simulink model "prueba_cinematica"  (Simulink 7.6)
settings: Solver=ode45  StartTime=0.0  StopTime=10.0  RelTol=1e-3
undefined symbols (not defined in the file or in its folder): phi0, psi0, theta0, x0, y0, z0
settings Model: Creator=pater  LastModifiedBy=pater

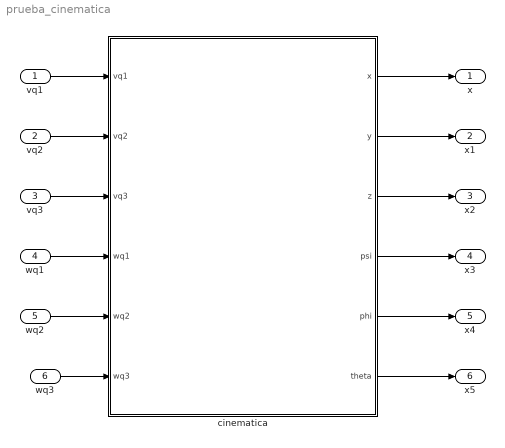
== system prueba_cinematica ==
  vq1 : Inport
  vq2 : Inport  Port=2
  vq3 : Inport  Port=3
  wq1 : Inport  Port=4
  wq2 : Inport  Port=5
  wq3 : Inport  Port=6
  cinematica : Subsystem
  x : Outport
  x1 : Outport  Port=2
  x2 : Outport  Port=3
  x3 : Outport  Port=4
  x4 : Outport  Port=5
  x5 : Outport  Port=6
  wires:
  vq1/1 -> cinematica/1(vq1)
  vq2/1 -> cinematica/2(vq2)
  vq3/1 -> cinematica/3(vq3)
  wq1/1 -> cinematica/4(wq1)
  wq2/1 -> cinematica/5(wq2)
  wq3/1 -> cinematica/6(wq3)
  cinematica/6(theta) -> x5/1
  cinematica/5(phi) -> x4/1
  cinematica/4(psi) -> x3/1
  cinematica/3(z) -> x2/1
  cinematica/2(y) -> x1/1
  cinematica/1(x) -> x/1

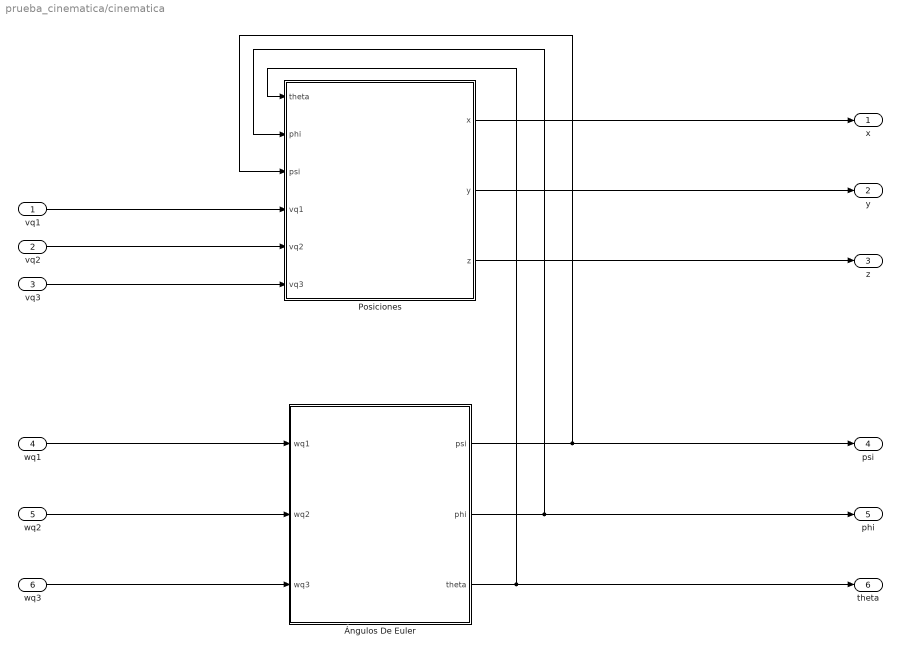
== system prueba_cinematica/cinematica ==
  vq1 : Inport
  vq2 : Inport  Port=2
  vq3 : Inport  Port=3
  wq1 : Inport  Port=4
  wq2 : Inport  Port=5
  wq3 : Inport  Port=6
  Posiciones : Subsystem
  Ángulos De Euler : Subsystem
  x : Outport
  y : Outport  Port=2
  z : Outport  Port=3
  psi : Outport  Port=4
  phi : Outport  Port=5
  theta : Outport  Port=6
  wires:
  Posiciones/1(x) -> x/1
  Posiciones/2(y) -> y/1
  Posiciones/3(z) -> z/1
  Ángulos De Euler/1(psi) -> psi/1, Posiciones/3(psi)
  Ángulos De Euler/2(phi) -> phi/1, Posiciones/2(phi)
  Ángulos De Euler/3(theta) -> theta/1, Posiciones/1(theta)
  vq1/1 -> Posiciones/4(vq1)
  vq2/1 -> Posiciones/5(vq2)
  vq3/1 -> Posiciones/6(vq3)
  wq1/1 -> Ángulos De Euler/1(wq1)
  wq2/1 -> Ángulos De Euler/2(wq2)
  wq3/1 -> Ángulos De Euler/3(wq3)

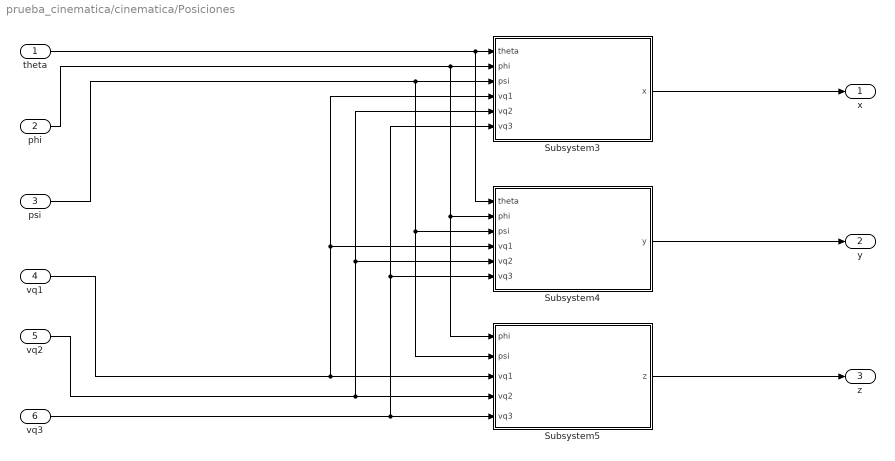
== system prueba_cinematica/cinematica/Posiciones ==
  theta : Inport
  phi : Inport  Port=2
  psi : Inport  Port=3
  vq1 : Inport  Port=4
  vq2 : Inport  Port=5
  vq3 : Inport  Port=6
  Subsystem3 : Subsystem
  Subsystem4 : Subsystem
  Subsystem5 : Subsystem
  x : Outport
  y : Outport  Port=2
  z : Outport  Port=3
  wires:
  Subsystem3/1(x) -> x/1
  Subsystem4/1(y) -> y/1
  Subsystem5/1(z) -> z/1
  vq3/1 -> Subsystem5/5(vq3), Subsystem4/6(vq3), Subsystem3/6(vq3)
  theta/1 -> Subsystem3/1(theta), Subsystem4/1(theta)
  phi/1 -> Subsystem3/2(phi), Subsystem4/2(phi), Subsystem5/1(phi)
  psi/1 -> Subsystem3/3(psi), Subsystem4/3(psi), Subsystem5/2(psi)
  vq2/1 -> Subsystem5/4(vq2), Subsystem4/5(vq2), Subsystem3/5(vq2)
  vq1/1 -> Subsystem5/3(vq1), Subsystem4/4(vq1), Subsystem3/4(vq1)

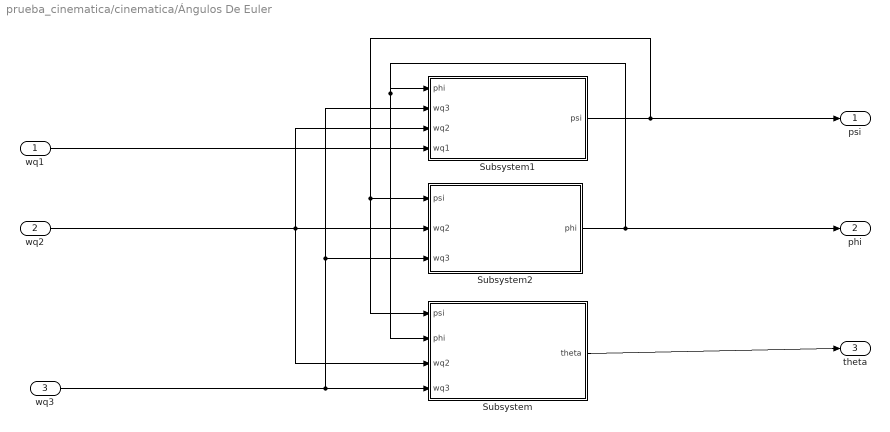
== system prueba_cinematica/cinematica/Ángulos De Euler ==
  wq1 : Inport
  wq2 : Inport  Port=2
  wq3 : Inport  Port=3
  Subsystem : Subsystem
  Subsystem1 : Subsystem
  Subsystem2 : Subsystem
  psi : Outport
  phi : Outport  Port=2
  theta : Outport  Port=3
  wires:
  Subsystem1/1(psi) -> psi/1, Subsystem/1(psi), Subsystem2/1(psi)
  Subsystem2/1(phi) -> phi/1, Subsystem/2(phi), Subsystem1/1(phi)
  Subsystem/1(theta) -> theta/1
  wq3/1 -> Subsystem/4(wq3), Subsystem2/3(wq3), Subsystem1/2(wq3)
  wq1/1 -> Subsystem1/4(wq1)
  wq2/1 -> Subsystem2/2(wq2), Subsystem1/3(wq2), Subsystem/3(wq2)

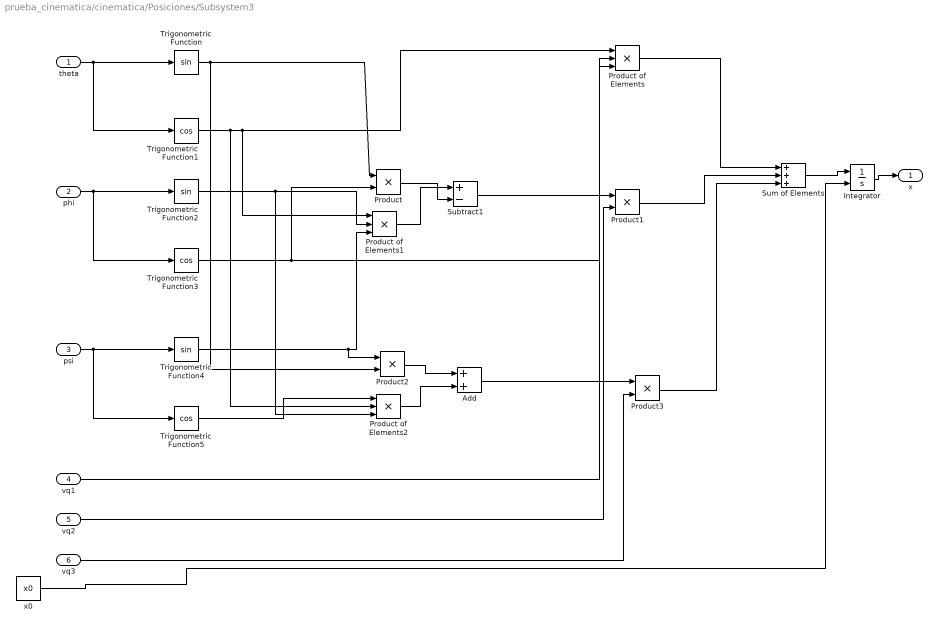
== system prueba_cinematica/cinematica/Posiciones/Subsystem3 ==
  theta : Inport
  phi : Inport  Port=2
  psi : Inport  Port=3
  vq1 : Inport  Port=4
  vq2 : Inport  Port=5
  vq3 : Inport  Port=6
  Add : Sum
  Integrator : Integrator  InitialConditionSource=external
  Product{,1..3} (4 alike) : Product  RndMeth=Zero
  Product of Elements : Product  Inputs=3
  Product of Elements1 : Product  Inputs=3
  Product of Elements2 : Product  Inputs=3
  Subtract1 : Sum  Inputs=+-
  Sum of Elements : Sum  Inputs=3
  Trigonometric Function : Trigonometry
  Trigonometric Function1 : Trigonometry  Operator=cos
  Trigonometric Function2 : Trigonometry
  Trigonometric Function3 : Trigonometry  Operator=cos
  Trigonometric Function4 : Trigonometry
  Trigonometric Function5 : Trigonometry  Operator=cos
  x0 : Constant  Value=x0
  x : Outport
  wires:
  theta/1 -> Trigonometric Function/1, Trigonometric Function1/1
  phi/1 -> Trigonometric Function2/1, Trigonometric Function3/1
  psi/1 -> Trigonometric Function4/1, Trigonometric Function5/1
  Trigonometric Function1/1 -> Product of Elements/1, Product of Elements1/1, Product of Elements2/2
  Trigonometric Function3/1 -> Product of Elements/2, Product/2
  vq1/1 -> Product of Elements/3
  Trigonometric Function/1 -> Product/1, Product2/2
  Trigonometric Function2/1 -> Product of Elements1/2, Product of Elements2/3
  Trigonometric Function4/1 -> Product of Elements1/3, Product2/1
  Subtract1/1 -> Product1/1
  vq2/1 -> Product1/2
  Product2/1 -> Add/1
  Product of Elements2/1 -> Add/2
  Trigonometric Function5/1 -> Product of Elements2/1
  Add/1 -> Product3/1
  vq3/1 -> Product3/2
  Product of Elements/1 -> Sum of Elements/1
  Product1/1 -> Sum of Elements/2
  Product3/1 -> Sum of Elements/3
  Sum of Elements/1 -> Integrator/1
  Integrator/1 -> x/1
  Product of Elements1/1 -> Subtract1/1
  Product/1 -> Subtract1/2
  x0/1 -> Integrator/2

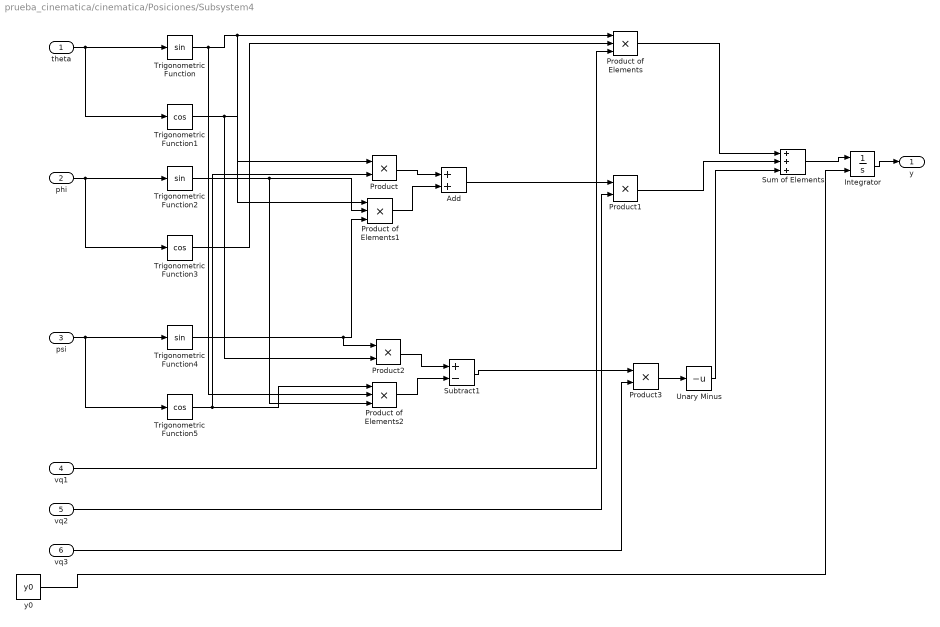
== system prueba_cinematica/cinematica/Posiciones/Subsystem4 ==
  theta : Inport
  phi : Inport  Port=2
  psi : Inport  Port=3
  vq1 : Inport  Port=4
  vq2 : Inport  Port=5
  vq3 : Inport  Port=6
  Add : Sum
  Integrator : Integrator  InitialConditionSource=external
  Product{,1..3} (4 alike) : Product  RndMeth=Zero
  Product of Elements : Product  Inputs=3
  Product of Elements1 : Product  Inputs=3
  Product of Elements2 : Product  Inputs=3
  Subtract1 : Sum  Inputs=+-
  Sum of Elements : Sum  Inputs=3
  Trigonometric Function : Trigonometry
  Trigonometric Function1 : Trigonometry  Operator=cos
  Trigonometric Function2 : Trigonometry
  Trigonometric Function3 : Trigonometry  Operator=cos
  Trigonometric Function4 : Trigonometry
  Trigonometric Function5 : Trigonometry  Operator=cos
  Unary Minus : UnaryMinus
  y0 : Constant  Value=y0
  y : Outport
  wires:
  theta/1 -> Trigonometric Function/1, Trigonometric Function1/1
  phi/1 -> Trigonometric Function2/1, Trigonometric Function3/1
  psi/1 -> Trigonometric Function4/1, Trigonometric Function5/1
  Trigonometric Function1/1 -> Product/1, Product2/2
  Trigonometric Function3/1 -> Product of Elements/2
  vq1/1 -> Product of Elements/3
  Trigonometric Function/1 -> Product of Elements/1, Product of Elements1/1, Product of Elements2/2
  Trigonometric Function2/1 -> Product of Elements1/2, Product of Elements2/3
  Trigonometric Function4/1 -> Product of Elements1/3, Product2/1
  Product/1 -> Add/1
  Product of Elements1/1 -> Add/2
  Add/1 -> Product1/1
  vq2/1 -> Product1/2
  Trigonometric Function5/1 -> Product of Elements2/1, Product/2
  Subtract1/1 -> Product3/1
  vq3/1 -> Product3/2
  Product of Elements/1 -> Sum of Elements/1
  Product1/1 -> Sum of Elements/2
  Product3/1 -> Unary Minus/1
  Sum of Elements/1 -> Integrator/1
  Integrator/1 -> y/1
  Unary Minus/1 -> Sum of Elements/3
  Product of Elements2/1 -> Subtract1/2
  Product2/1 -> Subtract1/1
  y0/1 -> Integrator/2

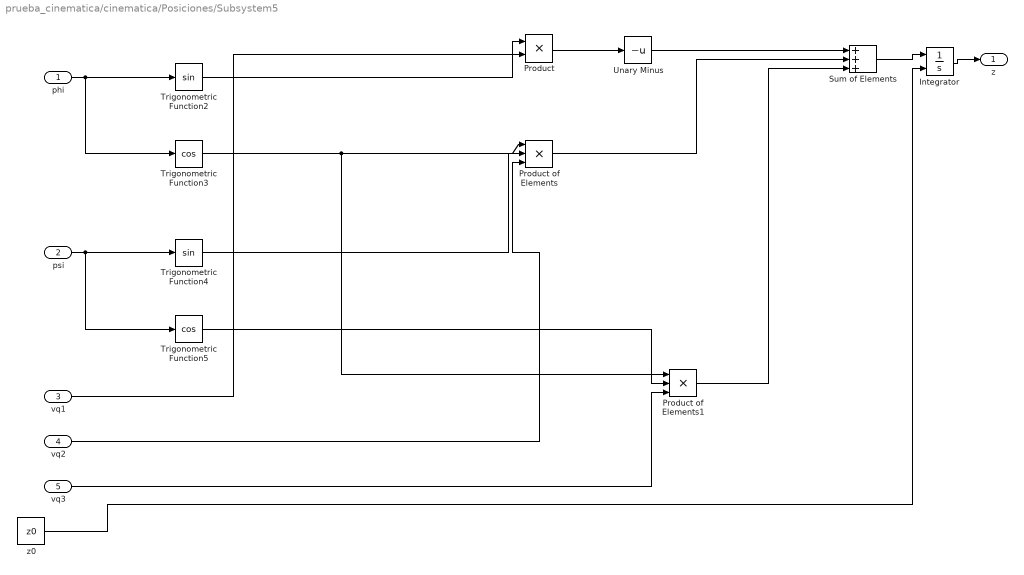
== system prueba_cinematica/cinematica/Posiciones/Subsystem5 ==
  phi : Inport
  psi : Inport  Port=2
  vq1 : Inport  Port=3
  vq2 : Inport  Port=4
  vq3 : Inport  Port=5
  Integrator : Integrator  InitialConditionSource=external
  Product : Product  RndMeth=Zero
  Product of Elements : Product  Inputs=3
  Product of Elements1 : Product  Inputs=3
  Sum of Elements : Sum  Inputs=3
  Trigonometric Function2 : Trigonometry
  Trigonometric Function3 : Trigonometry  Operator=cos
  Trigonometric Function4 : Trigonometry
  Trigonometric Function5 : Trigonometry  Operator=cos
  Unary Minus : UnaryMinus
  z0 : Constant  Value=z0
  z : Outport
  wires:
  phi/1 -> Trigonometric Function2/1, Trigonometric Function3/1
  psi/1 -> Trigonometric Function4/1, Trigonometric Function5/1
  Sum of Elements/1 -> Integrator/1
  Integrator/1 -> z/1
  Trigonometric Function2/1 -> Product/1
  vq1/1 -> Product/2
  Product/1 -> Unary Minus/1
  Trigonometric Function3/1 -> Product of Elements/1, Product of Elements1/1
  Trigonometric Function4/1 -> Product of Elements/2
  vq2/1 -> Product of Elements/3
  Trigonometric Function5/1 -> Product of Elements1/2
  vq3/1 -> Product of Elements1/3
  Product of Elements/1 -> Sum of Elements/2
  Product of Elements1/1 -> Sum of Elements/3
  Unary Minus/1 -> Sum of Elements/1
  z0/1 -> Integrator/2

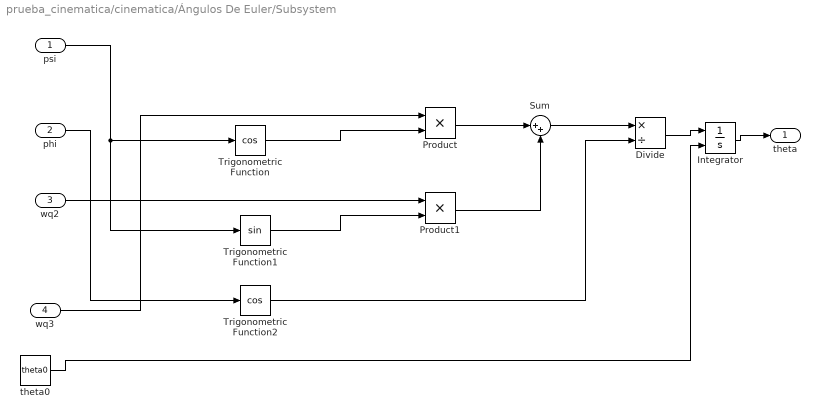
== system prueba_cinematica/cinematica/Ángulos De Euler/Subsystem ==
  psi : Inport
  phi : Inport  Port=2
  wq2 : Inport  Port=3
  wq3 : Inport  Port=4
  Divide : Product  Inputs=*/
  Integrator : Integrator  InitialConditionSource=external
  Product : Product  RndMeth=Zero
  Product1 : Product  RndMeth=Zero
  Sum : Sum  Inputs=|++
  Trigonometric Function : Trigonometry  Operator=cos
  Trigonometric Function1 : Trigonometry
  Trigonometric Function2 : Trigonometry  Operator=cos
  theta0 : Constant  Value=theta0
  theta : Outport
  wires:
  wq3/1 -> Product/1
  wq2/1 -> Product1/1
  Product/1 -> Sum/1
  Product1/1 -> Sum/2
  Sum/1 -> Divide/1
  Trigonometric Function2/1 -> Divide/2
  Divide/1 -> Integrator/1
  Trigonometric Function/1 -> Product/2
  Trigonometric Function1/1 -> Product1/2
  phi/1 -> Trigonometric Function2/1
  Integrator/1 -> theta/1
  psi/1 -> Trigonometric Function/1, Trigonometric Function1/1
  theta0/1 -> Integrator/2

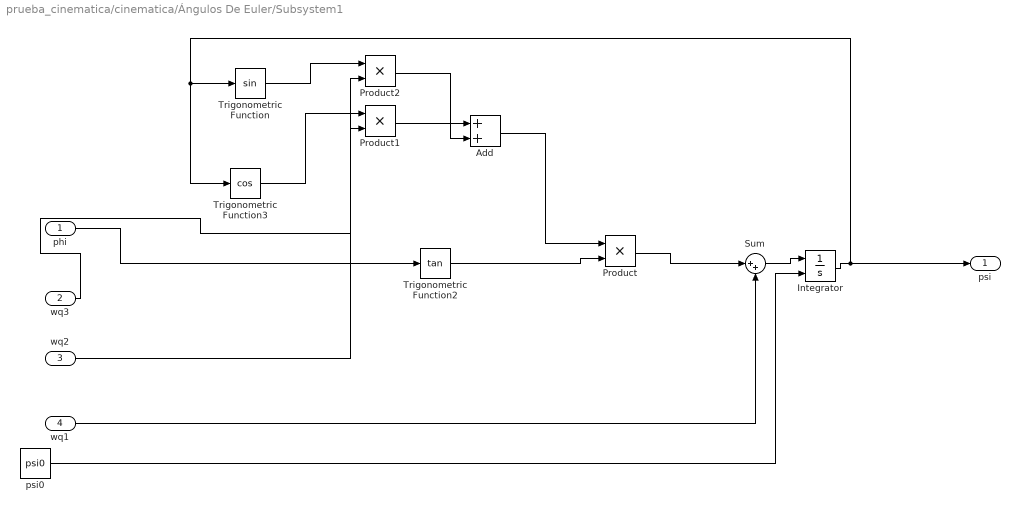
== system prueba_cinematica/cinematica/Ángulos De Euler/Subsystem1 ==
  phi : Inport
  wq3 : Inport  Port=2
  wq2 : Inport  Port=3
  wq1 : Inport  Port=4
  Add : Sum
  Integrator : Integrator  InitialConditionSource=external
  Product : Product  RndMeth=Zero
  Product1 : Product  RndMeth=Zero
  Product2 : Product  RndMeth=Zero
  Sum : Sum  Inputs=|++
  Trigonometric Function : Trigonometry
  Trigonometric Function2 : Trigonometry  Operator=tan
  Trigonometric Function3 : Trigonometry  Operator=cos
  psi0 : Constant  Value=psi0
  psi : Outport
  wires:
  Integrator/1 -> psi/1, Trigonometric Function3/1, Trigonometric Function/1
  Product/1 -> Sum/1
  phi/1 -> Trigonometric Function2/1
  Trigonometric Function2/1 -> Product/2
  wq3/1 -> Product1/2
  Trigonometric Function3/1 -> Product1/1
  Product1/1 -> Add/1
  Add/1 -> Product/1
  Trigonometric Function/1 -> Product2/1
  wq2/1 -> Product2/2
  Product2/1 -> Add/2
  wq1/1 -> Sum/2
  Sum/1 -> Integrator/1
  psi0/1 -> Integrator/2

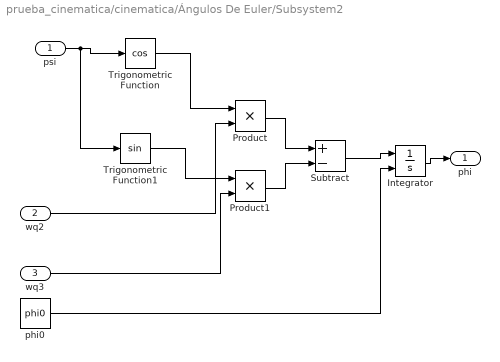
== system prueba_cinematica/cinematica/Ángulos De Euler/Subsystem2 ==
  psi : Inport
  wq2 : Inport  Port=2
  wq3 : Inport  Port=3
  Integrator : Integrator  InitialConditionSource=external
  Product : Product  RndMeth=Zero
  Product1 : Product  RndMeth=Zero
  Subtract : Sum  Inputs=+-
  Trigonometric Function : Trigonometry  Operator=cos
  Trigonometric Function1 : Trigonometry
  phi0 : Constant  Value=phi0
  phi : Outport
  wires:
  Integrator/1 -> phi/1
  Subtract/1 -> Integrator/1
  Product/1 -> Subtract/1
  Product1/1 -> Subtract/2
  Trigonometric Function/1 -> Product/1
  psi/1 -> Trigonometric Function/1, Trigonometric Function1/1
  Trigonometric Function1/1 -> Product1/1
  wq2/1 -> Product/2
  wq3/1 -> Product1/2
  phi0/1 -> Integrator/2
